simulink model "homing_ldm"  (R2017a)
settings: Solver=FixedStepAuto  StartTime=0.0  StopTime=inf  FixedStep=1e-3  RelTol=1e-3  EnableMultiTasking=on
libraries: xpcnilib x12, simulink x4
settings Model: SimulationMode=external  Creator=Davide  LastModifiedBy=Davide
settings SolverCC: EnableConcurrentExecution=on  ConcurrentTasks=on  AutoInsertRateTranBlk=on
settings DataIOCC: SaveFormat=StructureWithTime
settings OptimizationCC: BlockReduction=off  OptimizeBlockIOStorage=off  BufferReuse=off  GlobalBufferReuse=off  ExpressionFolding=off  LocalBlockOutputs=off
settings HardwareCC: ProdBitPerPointer=32  ProdBitPerSizeT=32  ProdBitPerPtrDiffT=32  ProdLargestAtomicFloat=None  ProdWordSize=32  ProdLongLongMode=on  ProdHWDeviceType=Generic->32-bit x86 compatible
settings RTWCC: SystemTargetFile=slrt.tlc  TemplateMakefile=slrt_default_tmf  Description=Simulink Real-Time  RTWCompilerOptimization=on
settings SimulinkRealTimeCC: xPCConcurrentTasks=on

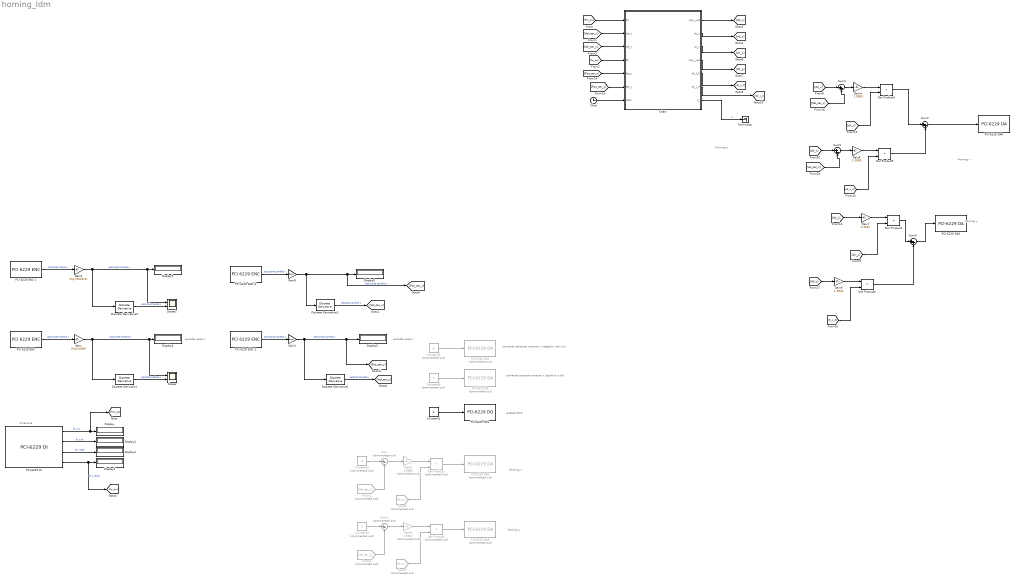
== system homing_ldm ==
  note: homing y
  note: Homing x
  note: enable P0.0
  note: comando tensione motore x (positivo a dx)
  note: comando tensione motore y (negativo vain su)
  note: Finecorsa
  note: encoder asse y
  note: encoder asse x
  note: Homing x
  note: homing y
  note: Homing x
  Chart : Stateflow chart  TreatAsAtomicUnit=on
  Clock : Clock
  Constant1 : Constant
  Constant2 : Constant  Commented=on  Value=-2
  Constant3 : Constant  Commented=on  Value=-2
  Constant4 : Constant  Commented=on
  Constant5 : Constant  Commented=on  Value=2
  Discrete Derivative{,1..3} (4 alike) : simulink/Discrete/Discrete Derivative  gainval=1.0  ICPrevScaledInput=0.0  OutMin=[]  OutMax=[]  OutDataType=fixdt(1, 16)  OutScaling=2^-10  DoSatur=off
  Display{,1..6,9} (8 alike) : Display
  Dot Product1 : DotProduct  Commented=on  InputSameDT=on  OutDataTypeStr=Inherit: Inherit via internal rule
  Dot Product2 : DotProduct  Commented=on  InputSameDT=on  OutDataTypeStr=Inherit: Inherit via internal rule
  Dot Product{3..6} (4 alike) : DotProduct  InputSameDT=on  OutDataTypeStr=Inherit: Inherit via internal rule
  From4 : From  Commented=on  GotoTag=Vel_car_x
  From5 : From  Commented=on  GotoTag=Fcx_sx
  From6 : From  Commented=on  GotoTag=Vel_car_y
  From7 : From  Commented=on  GotoTag=Fcy_dw
  Gain : Gain  Gain=2*pi/(4096)
  Gain1 : Gain  Gain=-5e-6
  Gain2 : Gain  Gain=2*pi/(1024*4)
  Gain3 : Gain  Gain=-5e-6
  Gain4 : Gain  Gain=1.0989
  Gain5 : Gain  Commented=on  Gain=1.0989
  Gain6 : Gain  Commented=on  Gain=1.5942
  Gain7 : Gain  Gain=1.5942
  Gain8 : Gain  Gain=1.0989
  Gain9 : Gain  Gain=1.5942
  "PCI 6229 ENC " : xpcnilib/Incremental Encoder/PCI 6229 ENC   channel=0  countMode=Quadrature Mode x4  initCount=0  reload=on  indexPhase=A low B low  filter=None  sampleTime=0.001  slot=[4 12]
      settings: SourceProductName=Simulink Real-Time  SourceProductBaseCode=XP
  PCI 6229 ENC 1 : xpcnilib/Incremental Encoder/PCI 6229 ENC   channel=1  countMode=Quadrature Mode x4  initCount=0  reload=on  indexPhase=A low B low  filter=None  sampleTime=0.001  slot=[4 12]
      settings: SourceProductName=Simulink Real-Time  SourceProductBaseCode=XP
  PCI 6229 ENC 2 : xpcnilib/Incremental Encoder/PCI 6229 ENC   channel=0  countMode=Quadrature Mode x4  initCount=0  reload=on  indexPhase=A low B low  filter=None  sampleTime=0.001  slot=[4 15]
      settings: SourceProductName=Simulink Real-Time  SourceProductBaseCode=XP
  PCI 6229 ENC 3 : xpcnilib/Incremental Encoder/PCI 6229 ENC   channel=1  countMode=Quadrature Mode x4  initCount=0  reload=on  indexPhase=A low B low  filter=None  sampleTime=0.001  slot=[4 15]
      settings: SourceProductName=Simulink Real-Time  SourceProductBaseCode=XP
  PCI-6229 DA : xpcnilib/D//A/M Series/PCI-6229 DA  Commented=on  channel=[1]  reset=[1]  initValue=[0]  sampletime=0.001  slot=[4 12]
      settings: SourceProductName=Simulink Real-Time  SourceProductBaseCode=XP
  PCI-6229 DA1 : xpcnilib/D//A/M Series/PCI-6229 DA  Commented=on  channel=[1]  reset=[1]  initValue=[0]  sampletime=0.001  slot=[4 15]
      settings: SourceProductName=Simulink Real-Time  SourceProductBaseCode=XP
  PCI-6229 DA2 : xpcnilib/D//A/M Series/PCI-6229 DA  Commented=on  channel=[1]  reset=[1]  initValue=[0]  sampletime=0.001  slot=[4 12]
      settings: SourceProductName=Simulink Real-Time  SourceProductBaseCode=XP
  PCI-6229 DA3 : xpcnilib/D//A/M Series/PCI-6229 DA  Commented=on  channel=[1]  reset=[1]  initValue=[0]  sampletime=0.001  slot=[4 15]
      settings: SourceProductName=Simulink Real-Time  SourceProductBaseCode=XP
  PCI-6229 DA4 : xpcnilib/D//A/M Series/PCI-6229 DA  channel=[1]  reset=[1]  initValue=[0]  sampletime=0.001  slot=[4 12]
      settings: SourceProductName=Simulink Real-Time  SourceProductBaseCode=XP
  PCI-6229 DA5 : xpcnilib/D//A/M Series/PCI-6229 DA  channel=[1]  reset=[1]  initValue=[0]  sampletime=0.001  slot=[4 15]
      settings: SourceProductName=Simulink Real-Time  SourceProductBaseCode=XP
  PCI-6229 DI : xpcnilib/Digital Input/M Series/PCI-6229 DI  channel=[4 5 6 7]  sampletime=0.001  slot=[4 12]
      settings: SourceProductName=Simulink Real-Time  SourceProductBaseCode=XP
  PCI-6229 DO1 : xpcnilib/Digital Output/M Series/PCI-6229 DO  channel=[1]  reset=[1]  initValue=[0]  sampletime=0.001  slot=[4 12]
      settings: SourceProductName=Simulink Real-Time  SourceProductBaseCode=XP
  Scope : Scope  NumInputPorts=2
  Scope2 : Scope  NumInputPorts=2
  Sum : Sum  Commented=on  Inputs=|+-
  Sum1 : Sum  Commented=on  Inputs=|+-
  Sum2 : Sum  Inputs=|++
  Sum3 : Sum  Inputs=|++
  Sum4 : Sum  Inputs=|+-
  Sum5 : Sum  Inputs=|+-
  Terminator : Terminator
  wires:
  PCI-6229 DI/1 -> [Fcx_sx], Display/1  "fc x sx"
  PCI-6229 DI/2 -> Display1/1  "fc x dx"
  PCI-6229 DI/3 -> Display2/1  "fc y high"
  PCI-6229 DI/4 -> [Fcy_dw], Display3/1  "fc y down"
  PCI 6229 ENC 1/1 -> Gain2/1  "pozione motore y"
  PCI 6229 ENC 3/1 -> Gain3/1  "posizione carrello x"
  PCI 6229 ENC 2/1 -> Gain1/1  "posizione carrello y"
  "PCI 6229 ENC "/1 -> Gain/1  "posizione motore x"
  Discrete Derivative/1 -> Scope/2  "velocità motore x"
  Discrete Derivative1/1 -> [Vel_car_y]  "velocità carrello y"
  Gain/1 -> Display4/1, Scope/1, Discrete Derivative/1  "posizione motore x"
  Gain1/1 -> [Pos_car_y], Display5/1, Discrete Derivative1/1  "posizione carrello y"
  Gain2/1 -> Scope2/1, Display9/1, Discrete Derivative2/1  "posizione motore y"
  Gain3/1 -> Discrete Derivative3/1, [Pos_car_x], Display6/1  "posizione carrello x"
  Constant1/1 -> PCI-6229 DO1/1
  Constant3/1 -> PCI-6229 DA1/1
  Discrete Derivative2/1 -> Scope2/2  "velocità motore y"
  Discrete Derivative3/1 -> [Vel_car_x]  "velocità carrello x"
  [Fcx_sx] -> Chart/1(fcx)
  [Vel_car_x] -> Chart/2(Vel_x)
  Chart/1(Vel_x_out) -> [dV_x]
  Constant2/1 -> Sum/1
  From4/1 -> Sum/2
  Sum/1 -> Gain5/1
  Gain5/1 -> Dot Product1/1
  Dot Product1/1 -> PCI-6229 DA2/1
  From5/1 -> Dot Product1/2
  Constant4/1 -> Sum1/1
  Gain6/1 -> Dot Product2/1
  Sum1/1 -> Gain6/1
  Dot Product2/1 -> PCI-6229 DA3/1
  From6/1 -> Sum1/2
  From7/1 -> Dot Product2/2
  Constant5/1 -> PCI-6229 DA/1
  [Fcy_dw] -> Chart/4(fcy)
  [Vel_car_y] -> Chart/3(Vel_y)
  Chart/2(ok_x) -> [ok_x]
  Chart/3(ok_y) -> [ok_y]
  Chart/4(Vel_y_out) -> [dV_y]
  [dV_y] -> Gain7/1
  Gain4/1 -> Dot Product3/1
  [ok_x] -> Dot Product3/2
  [ok_y] -> Dot Product4/2
  Gain7/1 -> Dot Product4/1
  Dot Product5/1 -> Sum2/2
  [ok_x_2] -> Dot Product5/2
  Gain8/1 -> Dot Product5/1
  Sum5/1 -> Gain8/1
  [Pos_car_x] -> Chart/5(Pos_x)
  Chart/5(ok_x_2) -> [ok_x_2]
  Dot Product3/1 -> Sum2/1
  Chart/6(ok_y_2) -> [ok_y_2]
  [Pos_car_y] -> Chart/6(Pos_y)
  [dV_y] -> Gain9/1
  Gain9/1 -> Dot Product6/1
  [ok_y_2] -> Dot Product6/2
  Dot Product6/1 -> Sum3/2
  Sum3/1 -> PCI-6229 DA5/1
  Dot Product4/1 -> Sum3/1
  Clock/1 -> Chart/7(clock)
  Chart/7(X_) -> Terminator/1  "X"
  [dV_x] -> Sum4/1
  Sum4/1 -> Gain4/1
  [Vel_car_x] -> Sum4/2
  [Vel_car_x] -> Sum5/2
  [dV_x] -> Sum5/1
  Sum2/1 -> PCI-6229 DA4/1

== stateflow chart homing_ldm/Chart ==
  state Homing
    state Homing_x
      entry:
      v_sp_x=-2.1;
      ok_x=1;
      ok_x_2=0;
      during:
      Vel_x_out=v_sp_x;
    state Homing_y
      entry:
      ok_x=0;
      v_sp_y=1.2;
      ok_y=1;
      during:
      Vel_y_out=v_sp_y-Vel_y;
    state Fine_homing1
      entry:
      ok_y=0;
      ok_x=0;
      a=Pos_x;
      ok_x_2=1;
      t1=clock;
      %X=0;
      %G_=0;
      %F_=0;
      %f_=0;
      during:
      t=clock-t1;
      %[G_,F_,f_]=Constant_Acceleration_ADIM_par(t,[1/3,1/3,1/3]);
      X_=Evaluate_Trajectory(t);
      Vel_x_out=X_;
      dx=Pos_x-a
    state Posizionamento_y
      entry:
      ok_x_2=0;
      ay=Pos_y;
      v_sp_y=-1.3;
      ok_y_2=1;
      during:
      Vel_y_out=v_sp_y-Vel_y;
      dy=abs(Pos_y-ay);
    state Fine
      entry:
      ok_y_2=0;
      ok_x_2=0;
    (default) -> Homing_x
    Homing_x -> Homing_y : [fcx==0]
    Homing_y -> Fine_homing1 : [fcy==0]
    Fine_homing1 -> Posizionamento_y : [dx>0.5]
    Posizionamento_y -> Fine : [dy>0.5]
  (default) -> Homing
  data: t1 local double; t local double; t function_input; X function_output; x function_input; par function_input; G function_output double; F function_output double; f function_output double; data2 function_output; fcx input; Vel_x_out output; Vel_x input; ok_x output; ok_y output; Vel_y input; Vel_y_out output; fcy input; Pos_x input; Pos_r_x local; dx local; ok_x_2 output; v_sp_x local; a local; v_sp_y local; ay local; Pos_y input; ok_y_2 output; dy local; clock input; X_ output double
  function X=Evaluate_Trajectory(t):
    | function X=Evaluate_Trajectory(t)
    | % parametri:
    | % t: tempo assolu
    | % h: spostamento richiesto
    | y=0;
    | yp=0;
    | ypp=0;
    | X=0;
    | 
    | h=0.5;
    | h0=0;
    | DT=[1/5 1/3 1/3 0]; %ta di ogni singolo ramo perche' composta
    | 
    | par = [1/3, 2/3];
    | 
    | 
    | DT1 = DT(1);
    | DT2 = DT(2);
    | DT3 = DT(3);
    | DT4 = DT(4);
    | 
    | T0 = 0;
    | T1 = T0 + DT1;
    | T2 = T1 + DT2;
    | T3 = T2 + DT3;
    | T4  = T3 + DT4;                  % Total time
    | 
    | if t >= T0 && t <= T1            % Interval N°1 
    |    td = DT1; %tempo di azionamento
    |    x = (t - T0)/td; %tempo adimensionale
    |    
    |    [G,F,f] = Constant_Acceleration_ADIM_par(x,par);
    |    y = h0 + G*h;
    |    yp = F * h/td;
    |    ypp = f * h/td^2;
    | end
    | 
    | if t > T1 && t <= T2             % Interval N°2 
    |    y = h0 + h;
    |    yp = 0;
    |    ypp = 0;
    | end
    | 
    | if t > T2 && t <= T3             % Interval N°3
    |    td = DT3;
    |    x = (t - T2)/td;
    |    
    |    [G,F,f] = Constant_Acceleration_ADIM_par(x,par);
    | 
    |    y = (h0 + h) - G*h;
    |    yp =  - (F * h/td);
    |    ypp = - (f * h/td^2);
    | end
    | 
    | if t > T3               % Interval N°4    
    |    y = h0;
    |    yp = 0;
    |    ypp = 0;  
    | end
    | Y = [y,yp,ypp];
    | X=yp;%pos, vel, acc
  function [G,F,f] = Constant_Acceleration_ADIM_par(x,par):
    | function [G,F,f] = Constant_Acceleration_ADIM_par(x,par)
    | % function [G,F,f] = Constant_Acceleration_ADIM_par(x,par)
    | % prof. Paolo Righettini
    | % Progettazione Funzionale di Sistemi Meccanici e Meccatronici
    | %
    | % x = t/td
    | % par(1) = adimensional time (start point at maximum velocity)
    | % par(2) = adimensional time (end point at maximum velocity)
    | % G = adimensionalized displacement
    | % F = adimensionalized velocity
    | % f = adimensionalized acceleration
    | G=0;
    | F=0;
    | f=0;
    | xv = par(1);
    | xw = par(2);
    |   
    | 
    | 
    | A = 2/(xv *(1-xv+xw));
    | B = 2/((1-xw)*(1-xv+xw));
    | 
    | if x>=0 & x<=xv
    |    f=A;
    |    F=A*x;
    |    G=.5*A*x^2;
    | elseif x>xv & x<xw
    |    f=0;
    |    F=A*xv;
    |    G=A*xv*(x-xv/2);
    | elseif x>=xw & x<=1
    |    f=-B;
    |    F=A*xv-B*(x-xw);
    |    G=A*xv*(x-xv/2)-B/2*(x-xw)^2;
    | end
  function data2=prova:
    | function data2=prova()
    | data2=0;
    | end
